simulink model "Compressor"  (R2022b)
settings: Solver=VariableStepAuto  StartTime=0.0  StopTime=200  RelTol=1e-3
settings Model: Creator=Crapon  LastModifiedBy=Crapon

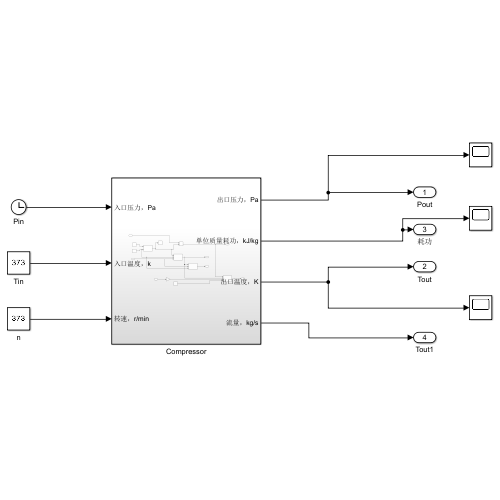
[thumbnail: Simulink's stored preview of the top-level diagram]
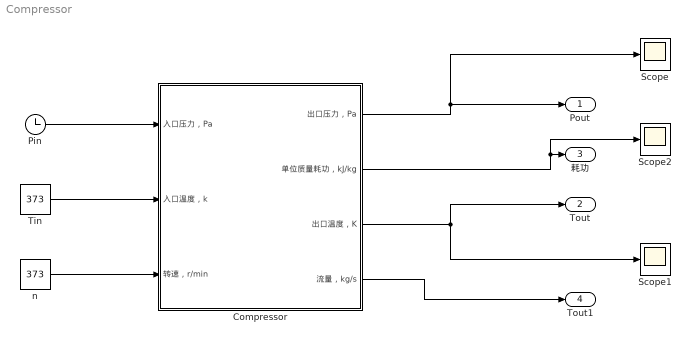
== system Compressor ==
  Compressor : Subsystem
  Pin : Clock
  Scope : Scope
  Scope1 : Scope
  Scope2 : Scope
  Tin : Constant  Value=373
  n : Constant  Value=373
  Pout : Outport
  Tout : Outport  Port=2
  耗功 : Outport  Port=3
  Tout1 : Outport  Port=4
  wires:
  Compressor/1(出口压力，Pa) -> Scope/1, Pout/1
  Compressor/3(出口温度，K) -> Tout/1, Scope1/1
  Compressor/2(单位质量耗功，kJ/kg) -> Scope2/1, 耗功/1
  Pin/1 -> Compressor/1(入口压力，Pa)
  Tin/1 -> Compressor/2(入口温度，k)
  Compressor/4(流量，kg/s) -> Tout1/1
  n/1 -> Compressor/3(转速，r/min)

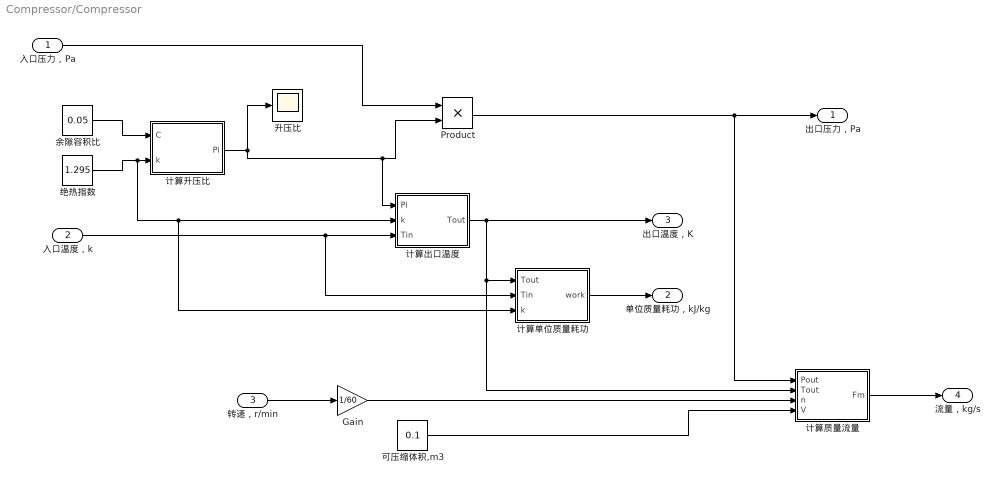
== system Compressor/Compressor ==
  入口压力，Pa : Inport
  入口温度，k : Inport  Port=2
  转速，r/min : Inport  Port=3
  Gain : Gain  Gain=1/60
  Product : Product
  余隙容积比 : Constant  Value=0.05
  升压比 : Scope
  可压缩体积,m3 : Constant  Value=0.1
  绝热指数 : Constant  Value=1.295
  计算出口温度 : MATLAB Function  TreatAsAtomicUnit=on
  计算升压比 : MATLAB Function  TreatAsAtomicUnit=on
  计算单位质量耗功 : MATLAB Function  TreatAsAtomicUnit=on
  计算质量流量 : MATLAB Function  TreatAsAtomicUnit=on
  出口压力，Pa : Outport
  单位质量耗功，kJ/kg : Outport  Port=2
  出口温度，K : Outport  Port=3
  流量，kg/s : Outport  Port=4
  wires:
  余隙容积比/1 -> 计算升压比/1(C)
  入口压力，Pa/1 -> Product/1
  绝热指数/1 -> 计算单位质量耗功/3(k), 计算出口温度/2(k), 计算升压比/2(k)
  Product/1 -> 计算质量流量/1(Pout), 出口压力，Pa/1
  计算单位质量耗功/1(work) -> 单位质量耗功，kJ/kg/1
  计算升压比/1(Pi) -> 计算出口温度/1(Pi), Product/2, 升压比/1
  入口温度，k/1 -> 计算单位质量耗功/2(Tin), 计算出口温度/3(Tin)
  计算出口温度/1(Tout) -> 出口温度，K/1, 计算质量流量/2(Tout), 计算单位质量耗功/1(Tout)
  计算质量流量/1(Fm) -> 流量，kg/s/1
  转速，r/min/1 -> Gain/1
  Gain/1 -> 计算质量流量/3(n)
  可压缩体积,m3/1 -> 计算质量流量/4(V)

== matlab function Compressor/计算出口温度 ==
  data: Pi input; Tout output; k input; Tin input
function Tout= fcn(Pi, k, Tin)

Tout=Tin*(Pi)^((k-1)/k);

== matlab function Compressor/计算单位质量耗功 ==
  data: Tout input; Tin input; k input; work output
function work= fcn(Tout,Tin,k)
Rg=0.189;
work=(k/(k-1))*Rg*(Tout-Tin);

== matlab function Compressor/计算升压比 ==
  data: C input; Pi output; k input
function Pi = fcn(C, k)

Pi =(1+1/C)^k;

== matlab function Compressor/计算质量流量 ==
  data: Pout input; Tout input; n input; V input; Fm output
function Fm = fcn(Pout, Tout,n, V)
a=refpropm('D','T',Tout,'P',Pout,'CO2');
Fm = a*V*n;
